simulink model "TransmissionMode_plausibility"  (R2024b)
settings: Solver=FixedStepAuto  StartTime=0.0  StopTime=20  FixedStep=0.1  RelTol=1e-3  EnableMultiTasking=on
settings Model: ExtModeTrigDuration=2  Creator=aayan  LastModifiedBy=aayan
settings SolverCC: AutoInsertRateTranBlk=on
settings OptimizationCC: EnhancedBackFolding=on  PassReuseOutputArgsAs=Individual arguments  ZeroExternalMemoryAtStartup=off  ZeroInternalMemoryAtStartup=off  MaxStackSize=64  OptimizeBlockOrder=speed  DifferentSizesBufferReuse=on  OptimizationCustomize=off  EfficientTunableParamExpr=on
settings DebuggingCC: ParameterTunabilityLossMsg=error
settings HardwareCC: ProdBitPerInt=16  ProdBitPerPointer=16  ProdBitPerSizeT=16  ProdBitPerPtrDiffT=16  ProdLargestAtomicFloat=None  ProdWordSize=8  ProdHWDeviceType=Atmel->AVR
settings SFSimCC: MATLABDynamicMemAlloc=off
settings RTWCC: Description=Embedded Coder  SystemTargetFile=ert.tlc  HardwareBoard=Arduino Uno  GenCodeOnly=on  TemplateMakefile=ert_default_tmf  Toolchain=Arduino AVR  BuildConfiguration=Faster Runs
settings CodeAppCC: ForceParamTrailComments=on  IgnoreCustomStorageClasses=off  OperatorAnnotations=on  SimulinkDataObjDesc=on  SFDataObjDesc=on  InsertBlockDesc=on
settings ERTTargetCC: SupportVariableSizeSignals=on  ExtModeTransport=3  ExtModeStaticAlloc=on  ExtModeAutomaticAllocSize=off  ExtModeStaticAllocSize=250  ExtModeMexFile=ext_xcp  ExtModeIntrfLevel=Level2 - Open  InlinedParameterPlacement=Hierarchical
settings ConfigComp: CovEnable=on  RecordCoverage=on  CovMetricSettings=dcmwe  CovModelRefEnable=on

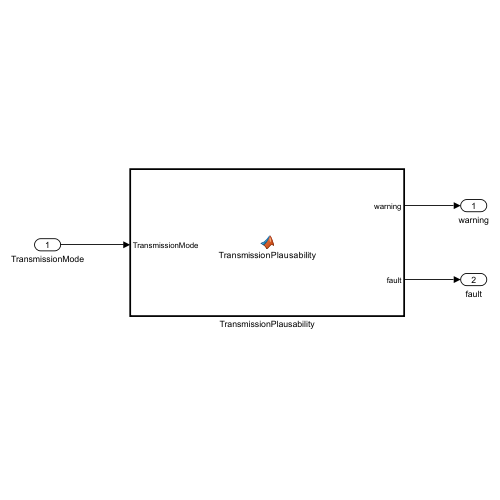
[thumbnail: Simulink's stored preview of the top-level diagram]
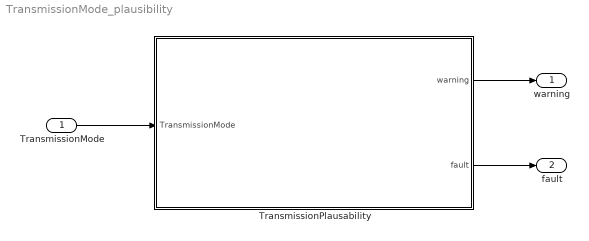
== system TransmissionMode_plausibility ==
  TransmissionMode : Inport  OutDataTypeStr=Enum: TransmissionState
  TransmissionPlausability : MATLAB Function  TreatAsAtomicUnit=on
  warning : Outport
  fault : Outport  Port=2
  wires:
  TransmissionPlausability/1(warning) -> warning/1
  TransmissionPlausability/2(fault) -> fault/1
  TransmissionMode/1 -> TransmissionPlausability/1(TransmissionMode)

== matlab function TransmissionMode_plausibility/TransmissionPlausability ==
  data: TransmissionMode input; warning output; fault output
function [warning, fault] = TransmissionPlausability(TransmissionMode)

% initialization
warning = boolean(0);
fault = boolean(0);

validModes = [ ...
    TransmissionState.Park, ...
    TransmissionState.Reverse, ...
    TransmissionState.Neutral, ...
    TransmissionState.Drive, ...
    TransmissionState.Brake ...
];

if ~any(TransmissionMode == validModes)
    warning = boolean(1);
    fault = boolean(1);
end
